simulink model "LQG"  (R2025b)
settings: Solver=ode23s  StartTime=0.0  StopTime=50.0  RelTol=1e-3
undefined symbols (not defined in the file): A, B, C, K_LQR_i, K_LQR_x, n, Qv, Rv, Ts, X0, x_ref
libraries: simulink x4, cstblocks x1
settings Model: Creator=salvo  LastModifiedBy=salvo

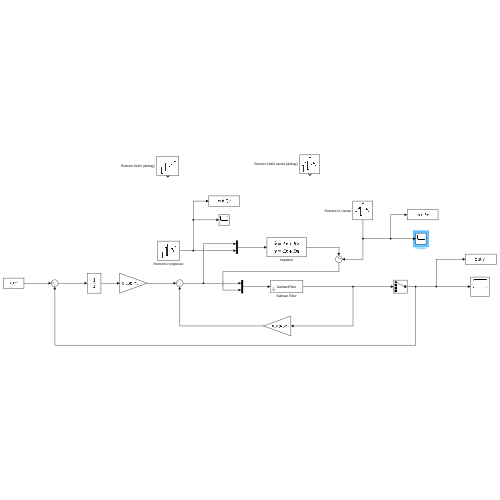
[thumbnail: Simulink's stored preview of the top-level diagram]
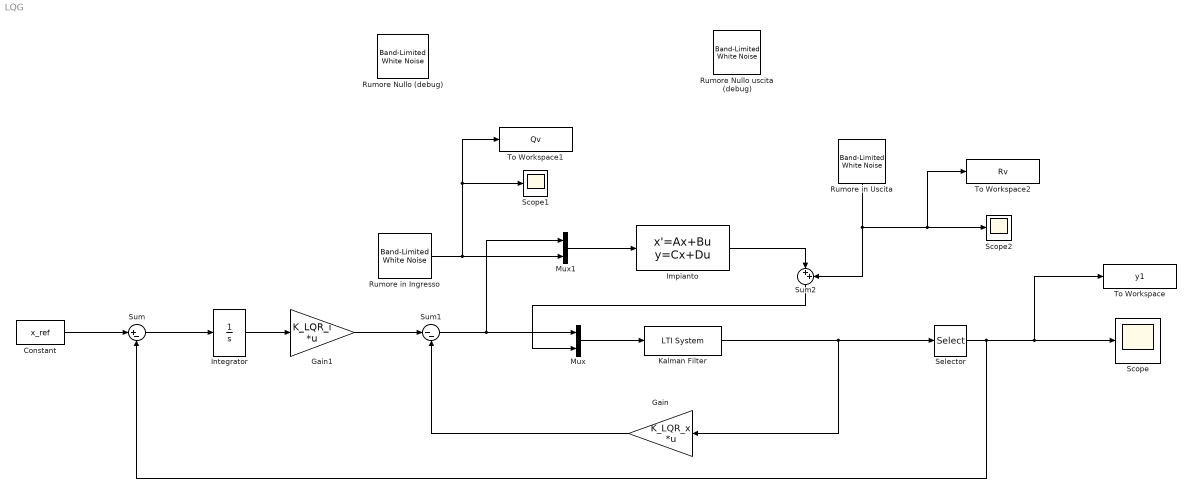
== system LQG ==
  Constant : Constant  Value=x_ref
  Gain : Gain  Gain=K_LQR_x  Multiplication=Matrix(K*u)
  Gain1 : Gain  Gain=K_LQR_i  Multiplication=Matrix(K*u)
  Impianto : StateSpace  A=A  B=[B eye(n)]  C=C  D=zeros(2,5)  InitialCondition=X0
  Integrator : Integrator
  Kalman Filter : cstblocks/LTI System  sys=KalmanFilter  IC=[]  PadeOrder=0
  Mux : Mux  Inputs=2
  Mux1 : Mux  Inputs=2
  Rumore Nullo (debug) : simulink/Sources/Band-Limited White Noise  Cov=diag(zeros(n))  Ts=Ts  seed=[23341]
  Rumore Nullo uscita (debug) : simulink/Sources/Band-Limited White Noise  Cov=0  Ts=Ts  seed=[23341]
  Rumore in Ingresso : simulink/Sources/Band-Limited White Noise  Cov=diag(Qv)  Ts=Ts  seed=[23341]
  Rumore in Uscita : simulink/Sources/Band-Limited White Noise  Cov=diag(Rv)  Ts=Ts  seed=[23341]
  Scope : Scope
      settings: ActiveDisplayYMinimum=-0.083793307434884945  ActiveDisplayYMaximum=0.39425931181451646
  Scope1 : Scope
      settings: ActiveDisplayYMinimum=-0.14505243452041064  ActiveDisplayYMaximum=0.11714619963355059
  Scope2 : Scope
      settings: ActiveDisplayYMinimum=-0.23148901620549184  ActiveDisplayYMaximum=0.27753401676508743  DataLoggingVariableName=ScopeData2
  Selector : Selector  InputPortWidth=4  IndexOptions=Index vector (dialog)  Indices=[1]  OutputSizes=1
  Sum : Sum  Inputs=|+-
  Sum1 : Sum  Inputs=|--
  Sum2 : Sum  Inputs=|++
  To Workspace : ToWorkspace  VariableName=y1  SaveFormat=Timeseries  SampleTime=-1
  To Workspace1 : ToWorkspace  VariableName=Qv  SaveFormat=Timeseries  SampleTime=-1
  To Workspace2 : ToWorkspace  VariableName=Rv  SaveFormat=Timeseries  SampleTime=-1
  wires:
  Gain1/1 -> Sum1/1
  Sum1/1 -> Mux/1, Mux1/1
  Gain/1 -> Sum1/2
  Integrator/1 -> Gain1/1
  Constant/1 -> Sum/1
  Sum/1 -> Integrator/1
  Selector/1 -> Scope/1, To Workspace/1, Sum/2
  Mux/1 -> Kalman Filter/1
  Kalman Filter/1 -> Gain/1, Selector/1
  Mux1/1 -> Impianto/1
  Rumore in Ingresso/1 -> Scope1/1, To Workspace1/1, Mux1/2
  Rumore in Uscita/1 -> Sum2/2, To Workspace2/1, Scope2/1
  Impianto/1 -> Sum2/1
  Sum2/1 -> Mux/2
